simulink model "ZynqBF_2tx_fpga"  (R2018b)
settings: Solver=FixedStepDiscrete  StartTime=0.0  StopTime=10.0  RelTol=1e-3
undefined symbols (not defined in the file or in its folder): gs1_i, gs1_q, gs2_i, gs2_q
libraries: hdlsllib x22, simulink x20, dsphdlfiltering x4
settings Model: DataTypeOverride=Off  Creator=jason  LastModifiedBy=jason
settings DataIOCC: SaveOutput=off  SaveTime=off
settings OptimizationCC: BlockReduction=off  ConditionallyExecuteInputs=off  DefaultParameterBehavior=Inlined
settings DebuggingCC: AlgebraicLoopMsg=error  SingleTaskRateTransMsg=error  ParameterPrecisionLossMsg=none  StrictBusMsg=ErrorOnBusTreatedAsVector
settings HardwareCC: ProdBitPerPointer=32  ProdBitPerSizeT=32  ProdBitPerPtrDiffT=32  ProdLargestAtomicFloat=None  ProdIntDivRoundTo=Undefined  ProdEndianess=Unspecified  ProdWordSize=32  ProdHWDeviceType=ASIC/FPGA->ASIC/FPGA  ProdEqTarget=off
settings SFSimCC: SimUseLocalCustomCode=off
settings RTWCC: RTWUseLocalCustomCode=off
settings CodeAppCC: StateflowObjectComments=on
settings GRTTargetCC: TargetLangStandard=C89/C90 (ANSI)

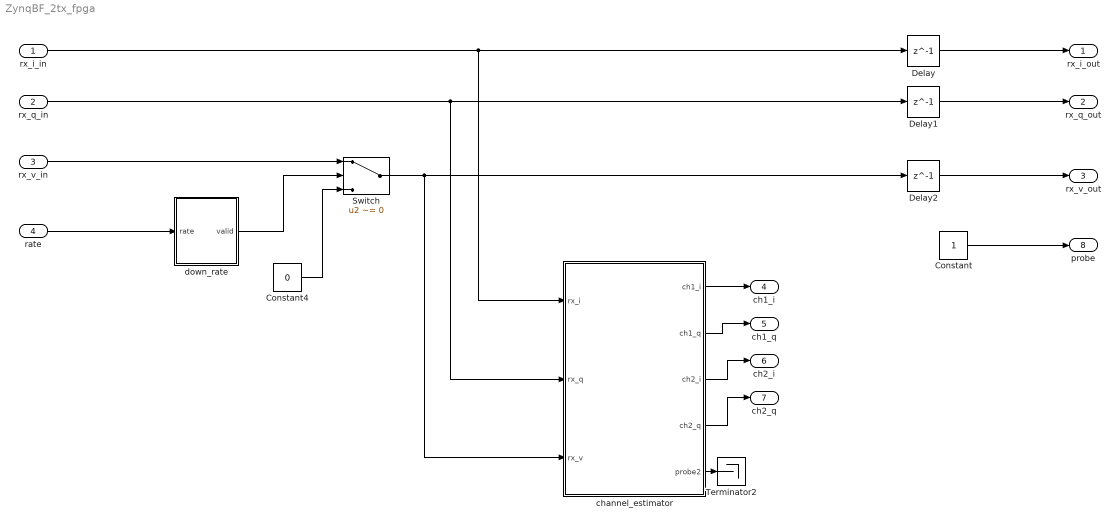
== system ZynqBF_2tx_fpga ==
  rx_i_in : Inport  OutDataTypeStr=fixdt(1,16,15)  SampleTime=1
  rx_q_in : Inport  Port=2  OutDataTypeStr=fixdt(1,16,15)  SampleTime=1
  rx_v_in : Inport  Port=3  OutDataTypeStr=boolean  SampleTime=1
  rate : Inport  Port=4  OutDataTypeStr=uint16  SampleTime=1
  Constant : Constant  OutDataTypeStr=uint16  SampleTime=-1
  Constant4 : Constant  Value=0  OutDataTypeStr=boolean  SampleTime=-1
  Delay : Delay  DelayLength=1
  Delay1 : Delay  DelayLength=1
  Delay2 : Delay  DelayLength=1
  Switch : Switch  Criteria=u2 ~= 0
  Terminator2 : Terminator
  channel_estimator : Subsystem  TreatAsAtomicUnit=on
  down_rate : Subsystem  TreatAsAtomicUnit=on
  rx_i_out : Outport  OutDataTypeStr=fixdt(1,16,15)
  rx_q_out : Outport  Port=2  OutDataTypeStr=fixdt(1,16,15)
  rx_v_out : Outport  Port=3  OutDataTypeStr=boolean  LockScale=on
  ch1_i : Outport  Port=4  OutDataTypeStr=fixdt(1,16,15)
  ch1_q : Outport  Port=5  OutDataTypeStr=fixdt(1,16,15)
  ch2_i : Outport  Port=6  OutDataTypeStr=fixdt(1,16,15)
  ch2_q : Outport  Port=7  OutDataTypeStr=fixdt(1,16,15)
  probe : Outport  Port=8
  wires:
  rate/1 -> down_rate/1(rate)
  rx_i_in/1 -> channel_estimator/1(rx_i), Delay/1
  rx_q_in/1 -> channel_estimator/2(rx_q), Delay1/1
  down_rate/1(valid) -> Switch/2
  rx_v_in/1 -> Switch/1
  Switch/1 -> channel_estimator/3(rx_v), Delay2/1
  Constant4/1 -> Switch/3
  Delay/1 -> rx_i_out/1
  Delay1/1 -> rx_q_out/1
  Delay2/1 -> rx_v_out/1
  channel_estimator/1(ch1_i) -> ch1_i/1
  channel_estimator/2(ch1_q) -> ch1_q/1
  channel_estimator/3(ch2_i) -> ch2_i/1
  channel_estimator/4(ch2_q) -> ch2_q/1
  channel_estimator/5(probe2) -> Terminator2/1
  Constant/1 -> probe/1

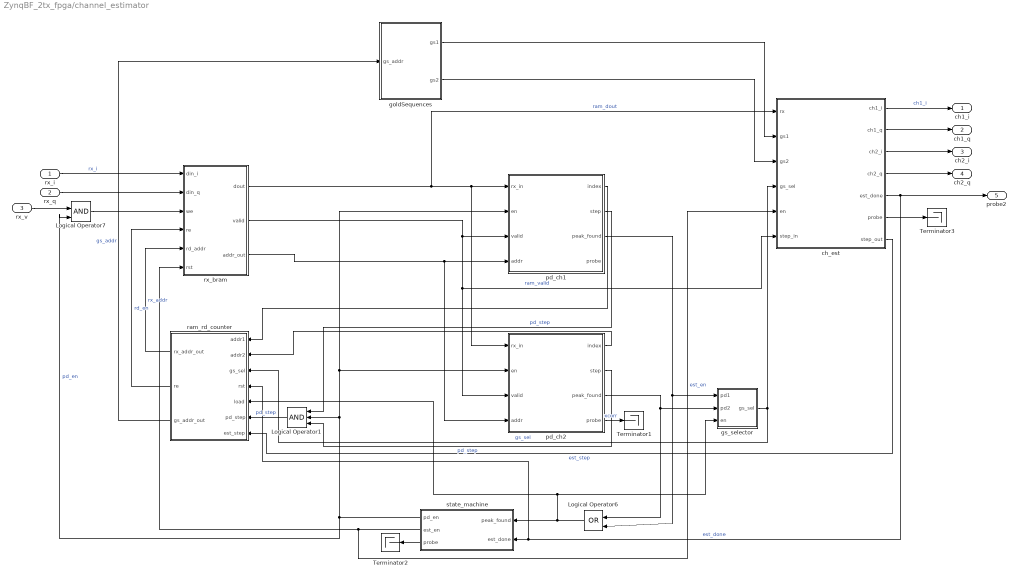
== system ZynqBF_2tx_fpga/channel_estimator ==
  rx_i : Inport
  rx_q : Inport  Port=2
  rx_v : Inport  Port=3
  Logical Operator1 : Logic  Inputs=3  IconShape=distinctive  AllPortsSameDT=off  OutDataTypeStr=boolean
  Logical Operator6 : Logic  Operator=OR  IconShape=distinctive  AllPortsSameDT=off  OutDataTypeStr=boolean
  Logical Operator7 : Logic  IconShape=distinctive  AllPortsSameDT=off  OutDataTypeStr=boolean
  Terminator1 : Terminator
  Terminator2 : Terminator
  Terminator3 : Terminator
  ch_est : Subsystem
  goldSequences : Subsystem
  gs_selector : Subsystem
  pd_ch1 : Subsystem
  pd_ch2 : Subsystem
  ram_rd_counter : Subsystem
  rx_bram : Subsystem
  state_machine : Subsystem
  ch1_i : Outport
  ch1_q : Outport  Port=2
  ch2_i : Outport  Port=3
  ch2_q : Outport  Port=4
  probe2 : Outport  Port=5
  wires:
  rx_q/1 -> rx_bram/2(din_q)
  rx_i/1 -> rx_bram/1(din_i)  "rx_i"
  Logical Operator7/1 -> rx_bram/3(we)
  pd_ch1/2(step) -> Logical Operator1/1  "pd_step"
  rx_bram/1(dout) -> ch_est/1(rx), pd_ch1/1(rx_in), pd_ch2/1(rx_in)  "ram_dout"
  goldSequences/1(gs1) -> ch_est/2(gs1)
  state_machine/1(pd_en) -> pd_ch1/2(en), pd_ch2/2(en), Logical Operator1/2, Logical Operator7/2  "pd_en"
  Logical Operator6/1 -> ram_rd_counter/5(load), gs_selector/3(en), state_machine/1(peak_found)
  ch_est/5(est_done) -> ram_rd_counter/4(rst), state_machine/2(est_done), probe2/1  "est_done"
  rx_v/1 -> Logical Operator7/1
  goldSequences/2(gs2) -> ch_est/3(gs2)
  pd_ch2/3(peak_found) -> Logical Operator6/1, gs_selector/2(pd2)
  pd_ch1/3(peak_found) -> Logical Operator6/2, gs_selector/1(pd1)
  gs_selector/1(gs_sel) -> ch_est/4(gs_sel), ram_rd_counter/3(gs_sel)  "gs_sel"
  ch_est/1(ch1_i) -> ch1_i/1  "ch1_i"
  ch_est/2(ch1_q) -> ch1_q/1
  ch_est/3(ch2_i) -> ch2_i/1
  ch_est/4(ch2_q) -> ch2_q/1
  rx_bram/2(valid) -> pd_ch1/3(valid), pd_ch2/3(valid), ch_est/6(step_in)  "ram_valid"
  Logical Operator1/1 -> ram_rd_counter/6(pd_step)  "pd_step"
  ram_rd_counter/1(rx_addr_out) -> rx_bram/5(rd_addr)  "rx_addr"
  ram_rd_counter/2(re) -> rx_bram/4(re)  "rd_en"
  state_machine/2(est_en) -> rx_bram/6(rst), ch_est/5(en)  "est_en"
  rx_bram/3(addr_out) -> pd_ch1/4(addr), pd_ch2/4(addr)
  ram_rd_counter/3(gs_addr_out) -> goldSequences/1(gs_addr)  "gs_addr"
  ch_est/7(step_out) -> ram_rd_counter/7(est_step)  "est_step"
  pd_ch2/2(step) -> Logical Operator1/3  "pd_step"
  pd_ch1/1(index) -> ram_rd_counter/1(addr1)
  pd_ch2/1(index) -> ram_rd_counter/2(addr2)
  pd_ch2/4(probe) -> Terminator1/1  "xcorr"
  state_machine/3(probe) -> Terminator2/1
  ch_est/6(probe) -> Terminator3/1

== system ZynqBF_2tx_fpga/down_rate ==
  rate : Inport
  HDL Counter : hdlsllib/Sources/HDL Counter  CountType=Free running  CountInit=0  CountStep=1  CountMax=25  CountFromType=Initial value  CountFrom=0  CountResetPort=on  CountLoadPort=off  CountEnbPort=off  CountDirPort=off  CountDataType=Unsigned  CountWordLen=8  CountFracLen=0  CountSampTime=1
      settings: SourceProductBaseCode=HD
  Relational Operator : RelationalOperator  OutDataTypeStr=boolean  RndMeth=Nearest
  valid : Outport
  wires:
  HDL Counter/1 -> Relational Operator/1
  Relational Operator/1 -> valid/1, HDL Counter/1
  rate/1 -> Relational Operator/2

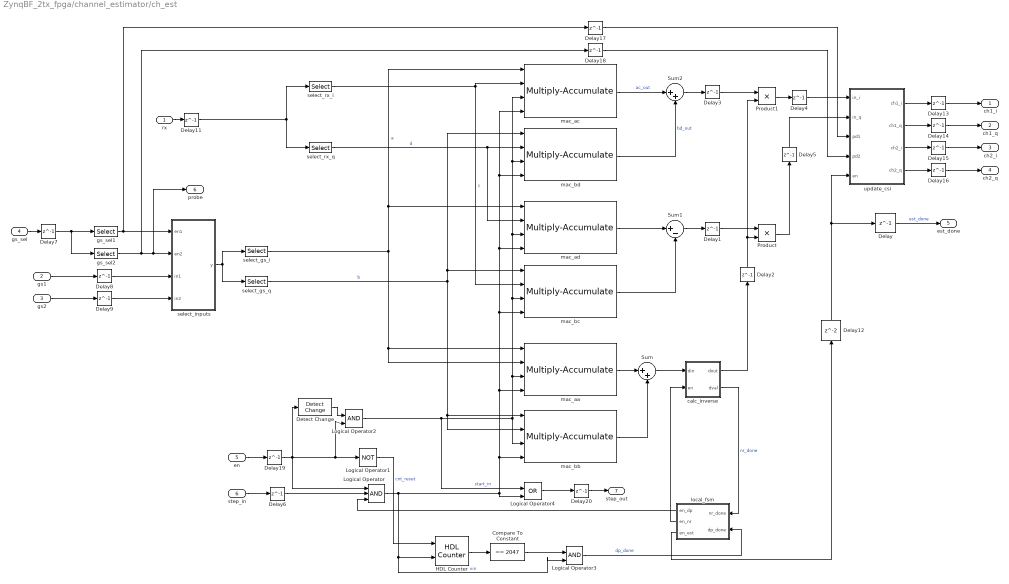
== system ZynqBF_2tx_fpga/channel_estimator/ch_est ==
  rx : Inport
  gs1 : Inport  Port=2
  gs2 : Inport  Port=3
  gs_sel : Inport  Port=4
  en : Inport  Port=5
  step_in : Inport  Port=6
  Compare To Constant : simulink/Logic and Bit Operations/Compare To Constant  relop===  const=2047  OutDataTypeStr=boolean
  Delay{,1..9,11,13..20} (19 alike) : Delay  DelayLength=1
  Delay12 : Delay
  Detect Change : simulink/Logic and Bit Operations/Detect Change  vinit=0  OutDataTypeStr=boolean
  HDL Counter : hdlsllib/Sources/HDL Counter  CountType=Count limited  CountInit=0  CountStep=1  CountMax=2047  CountFromType=Initial value  CountFrom=0  CountResetPort=on  CountLoadPort=off  CountEnbPort=on  CountDirPort=off  CountDataType=Unsigned  CountWordLen=16  CountFracLen=0  CountSampTime=-1
      settings: SourceProductBaseCode=HD
  Logical Operator : Logic  Inputs=3  IconShape=distinctive  AllPortsSameDT=off  OutDataTypeStr=boolean
  Logical Operator1 : Logic  Operator=NOT  IconShape=distinctive  AllPortsSameDT=off  OutDataTypeStr=boolean
  Logical Operator2 : Logic  IconShape=distinctive  AllPortsSameDT=off  OutDataTypeStr=boolean
  Logical Operator3 : Logic  IconShape=distinctive  AllPortsSameDT=off  OutDataTypeStr=boolean
  Logical Operator4 : Logic  Operator=OR  IconShape=distinctive  AllPortsSameDT=off  OutDataTypeStr=boolean
  Product : Product  OutDataTypeStr=fixdt(1,16,15)
  Product1 : Product  OutDataTypeStr=fixdt(1,16,15)
  Sum : Sum  Inputs=|++  OutDataTypeStr=fixdt(1,32,16)
  Sum1 : Sum  Inputs=|+-  OutDataTypeStr=fixdt(1,32,16)
  Sum2 : Sum  Inputs=|++  OutDataTypeStr=fixdt(1,32,16)
  calc_inverse : Subsystem
  gs_sel1 : Selector  IndexMode=Zero-based  InputPortWidth=2  IndexOptions=Index vector (dialog)  Indices=[0]  OutputSizes=1
  gs_sel2 : Selector  IndexMode=Zero-based  InputPortWidth=2  IndexOptions=Index vector (dialog)  Indices=[1]  OutputSizes=1
  local_fsm : Subsystem
  mac_aa : hdlsllib/HDL Operations/Multiply-Accumulate  opMode=Streaming - using Start and End ports  initValueSetting=Dialog  initValue=0  initValueSetting2=Dialog  initValue2=0  initValueSetting3=Dialog  initValue3=0  num_samples=2048  RndMeth2=Floor  RndMeth3=Floor  datatype2=fixdt(1,32,16)  datatype3=Inherit: Inherit via back propagation  validOut=off  endInandOut=off  startOut=off  countOut=off  dim=-1  DoSatur=off  parallel=off
      settings: SourceProductName=HDL Coder  SourceProductBaseCode=HD
  mac_ac : hdlsllib/HDL Operations/Multiply-Accumulate  opMode=Streaming - using Start and End ports  initValueSetting=Dialog  initValue=0  initValueSetting2=Dialog  initValue2=0  initValueSetting3=Dialog  initValue3=0  num_samples=2048  RndMeth2=Floor  RndMeth3=Floor  datatype2=fixdt(1,32,16)  datatype3=Inherit: Inherit via back propagation  validOut=off  endInandOut=off  startOut=off  countOut=off  dim=-1  DoSatur=off  parallel=off
      settings: SourceProductName=HDL Coder  SourceProductBaseCode=HD
  mac_ad : hdlsllib/HDL Operations/Multiply-Accumulate  opMode=Streaming - using Start and End ports  initValueSetting=Dialog  initValue=0  initValueSetting2=Dialog  initValue2=0  initValueSetting3=Dialog  initValue3=0  num_samples=2048  RndMeth2=Floor  RndMeth3=Floor  datatype2=fixdt(1,32,16)  datatype3=Inherit: Inherit via back propagation  validOut=off  endInandOut=off  startOut=off  countOut=off  dim=-1  DoSatur=off  parallel=off
      settings: SourceProductName=HDL Coder  SourceProductBaseCode=HD
  mac_bb : hdlsllib/HDL Operations/Multiply-Accumulate  opMode=Streaming - using Start and End ports  initValueSetting=Dialog  initValue=0  initValueSetting2=Dialog  initValue2=0  initValueSetting3=Dialog  initValue3=0  num_samples=2048  RndMeth2=Floor  RndMeth3=Floor  datatype2=fixdt(1,32,16)  datatype3=Inherit: Inherit via back propagation  validOut=off  endInandOut=off  startOut=off  countOut=off  dim=-1  DoSatur=off  parallel=off
      settings: SourceProductName=HDL Coder  SourceProductBaseCode=HD
  mac_bc : hdlsllib/HDL Operations/Multiply-Accumulate  opMode=Streaming - using Start and End ports  initValueSetting=Dialog  initValue=0  initValueSetting2=Dialog  initValue2=0  initValueSetting3=Dialog  initValue3=0  num_samples=2048  RndMeth2=Floor  RndMeth3=Floor  datatype2=fixdt(1,32,16)  datatype3=Inherit: Inherit via back propagation  validOut=off  endInandOut=off  startOut=off  countOut=off  dim=-1  DoSatur=off  parallel=off
      settings: SourceProductName=HDL Coder  SourceProductBaseCode=HD
  mac_bd : hdlsllib/HDL Operations/Multiply-Accumulate  opMode=Streaming - using Start and End ports  initValueSetting=Dialog  initValue=0  initValueSetting2=Dialog  initValue2=0  initValueSetting3=Dialog  initValue3=0  num_samples=2048  RndMeth2=Floor  RndMeth3=Floor  datatype2=fixdt(1,32,16)  datatype3=Inherit: Inherit via back propagation  validOut=off  endInandOut=off  startOut=off  countOut=off  dim=-1  DoSatur=off  parallel=off
      settings: SourceProductName=HDL Coder  SourceProductBaseCode=HD
  select_gs_i : Selector  IndexMode=Zero-based  InputPortWidth=2  IndexOptions=Index vector (dialog)  Indices=[0]  OutputSizes=1
  select_gs_q : Selector  IndexMode=Zero-based  InputPortWidth=2  IndexOptions=Index vector (dialog)  Indices=[1]  OutputSizes=1
  select_inputs : MATLAB Function  TreatAsAtomicUnit=on
  select_rx_i : Selector  IndexMode=Zero-based  InputPortWidth=2  IndexOptions=Index vector (dialog)  Indices=[0]  OutputSizes=1
  select_rx_q : Selector  IndexMode=Zero-based  InputPortWidth=2  IndexOptions=Index vector (dialog)  Indices=[1]  OutputSizes=1
  update_csi : Subsystem
  ch1_i : Outport
  ch1_q : Outport  Port=2
  ch2_i : Outport  Port=3
  ch2_q : Outport  Port=4
  est_done : Outport  Port=5
  probe : Outport  Port=6
  step_out : Outport  Port=7
  wires:
  gs_sel/1 -> Delay7/1
  select_rx_i/1 -> mac_bc/2, mac_ac/2  "c"
  select_rx_q/1 -> mac_ad/2, mac_bd/2  "d"
  Logical Operator/1 -> Logical Operator4/2, mac_ac/4, mac_bd/4, mac_ad/4, mac_bc/4, mac_aa/4, mac_bb/4, Logical Operator3/2, HDL Counter/2  "vin"
  gs1/1 -> Delay8/1
  gs2/1 -> Delay9/1
  select_inputs/1(y) -> select_gs_q/1, select_gs_i/1
  mac_ad/1 -> Sum1/1
  mac_bc/1 -> Sum1/2
  mac_ac/1 -> Sum2/1  "ac_out"
  mac_bd/1 -> Sum2/2  "bd_out"
  step_in/1 -> Delay6/1
  local_fsm/1(en_dp) -> Logical Operator/3
  Sum/1 -> calc_inverse/1(din)
  calc_inverse/2(dval) -> local_fsm/1(nr_done)  "nr_done"
  local_fsm/2(en_nr) -> calc_inverse/2(en)
  calc_inverse/1(dout) -> Delay2/1
  Sum1/1 -> Delay1/1
  Sum2/1 -> Delay3/1
  local_fsm/3(en_est) -> Delay12/1
  Product1/1 -> Delay4/1
  Product/1 -> Delay5/1
  update_csi/1(ch1_i) -> Delay13/1
  update_csi/2(ch1_q) -> Delay14/1
  update_csi/3(ch2_i) -> Delay15/1
  update_csi/4(ch2_q) -> Delay16/1
  Delay/1 -> est_done/1  "est_done"
  rx/1 -> Delay11/1
  Delay11/1 -> select_rx_i/1, select_rx_q/1
  Delay2/1 -> Product1/2, Product/2
  Delay1/1 -> Product/1
  Delay3/1 -> Product1/1
  Delay4/1 -> update_csi/1(in_i)
  Delay5/1 -> update_csi/2(in_q)
  Delay6/1 -> Logical Operator/2
  Delay8/1 -> select_inputs/3(in1)
  Delay9/1 -> select_inputs/4(in2)
  Delay12/1 -> Delay/1, update_csi/5(en)
  Delay13/1 -> ch1_i/1
  Delay14/1 -> ch1_q/1
  Delay15/1 -> ch2_i/1
  Delay16/1 -> ch2_q/1
  Delay7/1 -> gs_sel2/1, gs_sel1/1
  gs_sel2/1 -> Delay18/1, probe/1, select_inputs/2(en2)
  gs_sel1/1 -> Delay17/1, select_inputs/1(en1)
  Delay17/1 -> update_csi/3(pd1)
  Delay18/1 -> update_csi/4(pd2)
  select_gs_i/1 -> mac_aa/1, mac_aa/2, mac_ac/1, mac_ad/1  "a"
  select_gs_q/1 -> mac_bb/2, mac_bb/1, mac_bd/1, mac_bc/1  "b"
  en/1 -> Delay19/1
  Logical Operator1/1 -> HDL Counter/1  "cnt_reset"
  Delay19/1 -> Logical Operator/1, Detect Change/1, Logical Operator2/2, Logical Operator1/1
  Detect Change/1 -> Logical Operator2/1
  Logical Operator2/1 -> Logical Operator4/1, mac_bb/3, mac_aa/3, mac_bc/3, mac_ad/3, mac_bd/3, mac_ac/3  "start_in"
  HDL Counter/1 -> Compare To Constant/1
  mac_aa/1 -> Sum/1
  mac_bb/1 -> Sum/2
  Delay20/1 -> step_out/1
  Compare To Constant/1 -> Logical Operator3/1
  Logical Operator3/1 -> local_fsm/2(dp_done)  "dp_done"
  Logical Operator4/1 -> Delay20/1

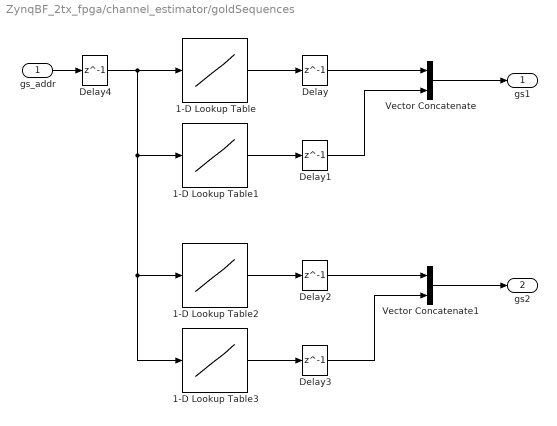
== system ZynqBF_2tx_fpga/channel_estimator/goldSequences ==
  gs_addr : Inport
  1-D Lookup Table : Lookup_n-D  NumberOfTableDimensions=1  LookupTableObject=''  BreakpointsForDimension1=[0:2047]  BreakpointsForDimension1FirstPoint=10  BreakpointsForDimension2FirstPoint=10  BreakpointsForDimension1Spacing=12  BreakpointsForDimension2Spacing=12  IndexSearchMethod=Evenly spaced points  Table=gs1_i  InterpMethod=Flat  DiagnosticForOutOfRangeInput=Error  InternalRulePriority=Speed  OutDataTypeStr=fixdt(1,16,15)  RndMeth=Simplest  InputSameDT=on
  1-D Lookup Table1 : Lookup_n-D  NumberOfTableDimensions=1  LookupTableObject=''  BreakpointsForDimension1=[0:2047]  BreakpointsForDimension1FirstPoint=10  BreakpointsForDimension2FirstPoint=10  BreakpointsForDimension1Spacing=12  BreakpointsForDimension2Spacing=12  IndexSearchMethod=Evenly spaced points  Table=gs1_q  InterpMethod=Flat  DiagnosticForOutOfRangeInput=Error  InternalRulePriority=Speed  OutDataTypeStr=fixdt(1,16,15)  RndMeth=Simplest  InputSameDT=on
  1-D Lookup Table2 : Lookup_n-D  NumberOfTableDimensions=1  LookupTableObject=''  BreakpointsForDimension1=[0:2047]  BreakpointsForDimension1FirstPoint=10  BreakpointsForDimension2FirstPoint=10  BreakpointsForDimension1Spacing=12  BreakpointsForDimension2Spacing=12  IndexSearchMethod=Evenly spaced points  Table=gs2_i  InterpMethod=Flat  DiagnosticForOutOfRangeInput=Error  InternalRulePriority=Speed  OutDataTypeStr=fixdt(1,16,15)  RndMeth=Simplest  InputSameDT=on
  1-D Lookup Table3 : Lookup_n-D  NumberOfTableDimensions=1  LookupTableObject=''  BreakpointsForDimension1=[0:2047]  BreakpointsForDimension1FirstPoint=10  BreakpointsForDimension2FirstPoint=10  BreakpointsForDimension1Spacing=12  BreakpointsForDimension2Spacing=12  IndexSearchMethod=Evenly spaced points  Table=gs2_q  InterpMethod=Flat  DiagnosticForOutOfRangeInput=Error  InternalRulePriority=Speed  OutDataTypeStr=fixdt(1,16,15)  RndMeth=Simplest  InputSameDT=on
  Delay{,1..4} (5 alike) : Delay  DelayLength=1
  Vector Concatenate : Concatenate
  Vector Concatenate1 : Concatenate
  gs1 : Outport
  gs2 : Outport  Port=2
  wires:
  1-D Lookup Table/1 -> Delay/1
  1-D Lookup Table1/1 -> Delay1/1
  1-D Lookup Table3/1 -> Delay3/1
  1-D Lookup Table2/1 -> Delay2/1
  Vector Concatenate/1 -> gs1/1
  Vector Concatenate1/1 -> gs2/1
  Delay/1 -> Vector Concatenate/1
  Delay1/1 -> Vector Concatenate/2
  Delay2/1 -> Vector Concatenate1/1
  Delay3/1 -> Vector Concatenate1/2
  gs_addr/1 -> Delay4/1
  Delay4/1 -> 1-D Lookup Table3/1, 1-D Lookup Table2/1, 1-D Lookup Table1/1, 1-D Lookup Table/1

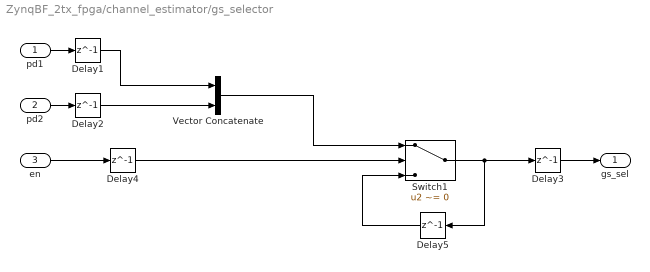
== system ZynqBF_2tx_fpga/channel_estimator/gs_selector ==
  pd1 : Inport
  pd2 : Inport  Port=2
  en : Inport  Port=3
  Delay{1..5} (5 alike) : Delay  DelayLength=1
  Switch1 : Switch  Criteria=u2 ~= 0
  Vector Concatenate : Concatenate
  gs_sel : Outport
  wires:
  pd2/1 -> Delay2/1
  en/1 -> Delay4/1
  pd1/1 -> Delay1/1
  Delay2/1 -> Vector Concatenate/2
  Delay1/1 -> Vector Concatenate/1
  Delay3/1 -> gs_sel/1
  Switch1/1 -> Delay3/1, Delay5/1
  Delay4/1 -> Switch1/2
  Vector Concatenate/1 -> Switch1/1
  Delay5/1 -> Switch1/3

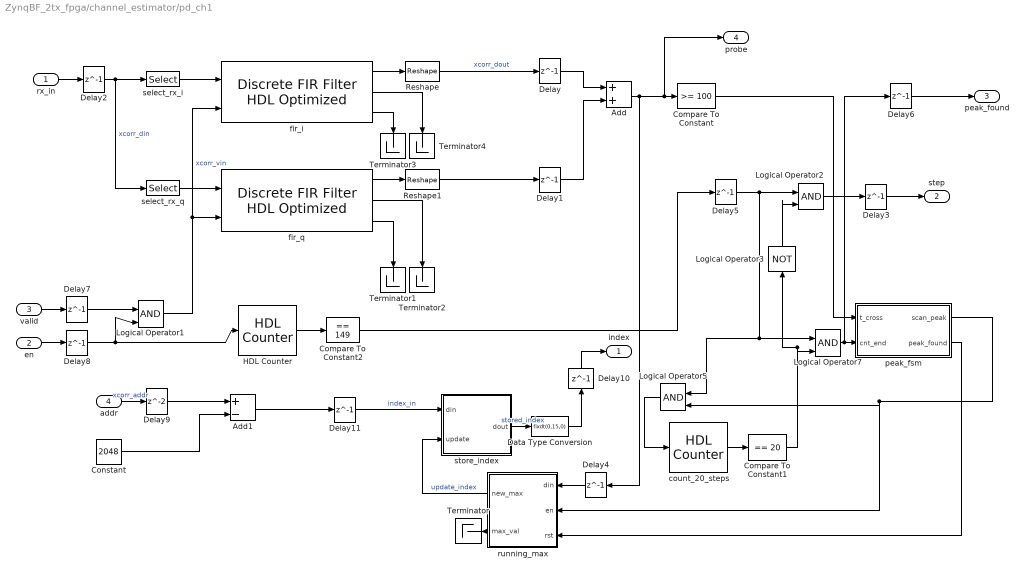
== system ZynqBF_2tx_fpga/channel_estimator/pd_ch1 ==
  rx_in : Inport
  en : Inport  Port=2
  valid : Inport  Port=3
  addr : Inport  Port=4
  Add : Sum  OutDataTypeStr=fixdt(1,32,16)
  Add1 : Sum  Inputs=+-  OutDataTypeStr=int16
  Compare To Constant : simulink/Logic and Bit Operations/Compare To Constant  relop=>=  const=100  OutDataTypeStr=boolean
  Compare To Constant1 : simulink/Logic and Bit Operations/Compare To Constant  relop===  const=20  OutDataTypeStr=boolean
  Compare To Constant2 : simulink/Logic and Bit Operations/Compare To Constant  relop===  const=149  OutDataTypeStr=boolean
  Constant : Constant  Value=2048  OutDataTypeStr=uint16  SampleTime=-1
  Data Type Conversion : DataTypeConversion  OutDataTypeStr=fixdt(0,15,0)
  Delay{,1..8,10..11} (11 alike) : Delay  DelayLength=1
  Delay9 : Delay
  HDL Counter : hdlsllib/Sources/HDL Counter  CountType=Count limited  CountInit=0  CountStep=1  CountMax=149  CountFromType=Initial value  CountFrom=0  CountResetPort=off  CountLoadPort=off  CountEnbPort=on  CountDirPort=off  CountDataType=Unsigned  CountWordLen=8  CountFracLen=0  CountSampTime=1
      settings: SourceProductBaseCode=HD
  Logical Operator{1..2,5,7} (4 alike) : Logic  IconShape=distinctive  AllPortsSameDT=off  OutDataTypeStr=boolean
  Logical Operator3 : Logic  Operator=NOT  IconShape=distinctive  AllPortsSameDT=off  OutDataTypeStr=boolean
  Reshape : Reshape
  Reshape1 : Reshape
  Terminator{,1..4} (5 alike) : Terminator
  count_20_steps : hdlsllib/Sources/HDL Counter  CountType=Count limited  CountInit=0  CountStep=1  CountMax=20  CountFromType=Initial value  CountFrom=0  CountResetPort=off  CountLoadPort=off  CountEnbPort=on  CountDirPort=off  CountDataType=Unsigned  CountWordLen=8  CountFracLen=0  CountSampTime=1
      settings: SourceProductBaseCode=HD
  fir_i : dsphdlfiltering/Discrete FIR Filter HDL Optimized  Numerator=fliplr(gs1_i')  FilterStructure=Direct form systolic  Sharing=on  SharingFactor=128  SimulateUsing=Code generation  roundingMode=Floor  overflowMode=off  CoefficientsDataTypeStr=Inherit: Same word length as input  CoefficientsMin=[]  CoefficientsMax=[]  OutputMin=[]  OutputMax=[]  ResetInputPort=off  HDLGlobalReset=off
      settings: SourceProductName=DSP System Toolbox  SourceProductBaseCode=DS
  fir_q : dsphdlfiltering/Discrete FIR Filter HDL Optimized  Numerator=fliplr(gs1_q')  FilterStructure=Direct form systolic  Sharing=on  SharingFactor=128  SimulateUsing=Code generation  roundingMode=Floor  overflowMode=off  CoefficientsDataTypeStr=Inherit: Same word length as input  CoefficientsMin=[]  CoefficientsMax=[]  OutputMin=[]  OutputMax=[]  ResetInputPort=off  HDLGlobalReset=off
      settings: SourceProductName=DSP System Toolbox  SourceProductBaseCode=DS
  peak_fsm : Subsystem
  running_max : Subsystem
  select_rx_i : Selector  IndexMode=Zero-based  InputPortWidth=2  IndexOptions=Index vector (dialog)  Indices=[0]  OutputSizes=1
  select_rx_q : Selector  IndexMode=Zero-based  InputPortWidth=2  IndexOptions=Index vector (dialog)  Indices=[1]  OutputSizes=1
  store_index : Subsystem
  index : Outport
  step : Outport  Port=2
  peak_found : Outport  Port=3
  probe : Outport  Port=4
  wires:
  Data Type Conversion/1 -> Delay10/1
  rx_in/1 -> Delay2/1
  fir_i/1 -> Reshape/1
  Reshape1/1 -> Delay1/1
  Delay1/1 -> Add/2
  Delay/1 -> Add/1
  Add/1 -> probe/1, Compare To Constant/1, Delay4/1
  Compare To Constant/1 -> peak_fsm/1(t_cross)
  Compare To Constant2/1 -> Delay5/1
  peak_fsm/1(scan_peak) -> running_max/2(en), Logical Operator5/2
  Logical Operator5/1 -> count_20_steps/1
  count_20_steps/1 -> Compare To Constant1/1
  Compare To Constant1/1 -> Logical Operator3/1, Logical Operator7/2
  Logical Operator7/1 -> Delay6/1, peak_fsm/2(cnt_end)
  peak_fsm/2(peak_found) -> running_max/3(rst)
  Delay4/1 -> running_max/1(din)
  running_max/2(max_val) -> Terminator/1
  en/1 -> Delay8/1
  Delay5/1 -> Logical Operator2/1, Logical Operator5/1, Logical Operator7/1
  Delay6/1 -> peak_found/1
  Reshape/1 -> Delay/1  "xcorr_dout"
  HDL Counter/1 -> Compare To Constant2/1
  fir_q/1 -> Reshape1/1
  valid/1 -> Delay7/1
  Logical Operator1/1 -> fir_i/2, fir_q/2  "xcorr_vin"
  Delay7/1 -> Logical Operator1/1
  Delay8/1 -> Logical Operator1/2, HDL Counter/1
  addr/1 -> Delay9/1  "xcorr_addr"
  Constant/1 -> Add1/2
  Delay9/1 -> Add1/1
  Add1/1 -> Delay11/1
  running_max/1(new_max) -> store_index/2(update)  "update_index"
  Delay11/1 -> store_index/1(din)  "index_in"
  store_index/1(dout) -> Data Type Conversion/1  "stored_index"
  Delay10/1 -> index/1
  Delay2/1 -> select_rx_q/1, select_rx_i/1  "xcorr_din"
  select_rx_i/1 -> fir_i/1
  select_rx_q/1 -> fir_q/1
  Logical Operator2/1 -> Delay3/1
  Logical Operator3/1 -> Logical Operator2/2
  Delay3/1 -> step/1
  fir_q/3 -> Terminator1/1
  fir_q/2 -> Terminator2/1
  fir_i/3 -> Terminator3/1
  fir_i/2 -> Terminator4/1

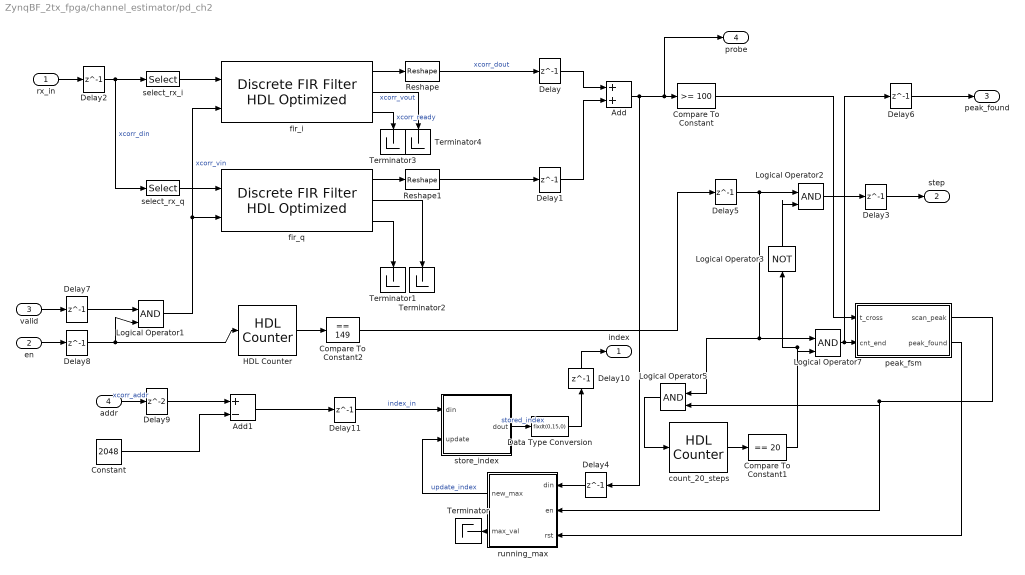
== system ZynqBF_2tx_fpga/channel_estimator/pd_ch2 ==
  rx_in : Inport
  en : Inport  Port=2
  valid : Inport  Port=3
  addr : Inport  Port=4
  Add : Sum  OutDataTypeStr=fixdt(1,32,16)
  Add1 : Sum  Inputs=+-  OutDataTypeStr=int16
  Compare To Constant : simulink/Logic and Bit Operations/Compare To Constant  relop=>=  const=100  OutDataTypeStr=boolean
  Compare To Constant1 : simulink/Logic and Bit Operations/Compare To Constant  relop===  const=20  OutDataTypeStr=boolean
  Compare To Constant2 : simulink/Logic and Bit Operations/Compare To Constant  relop===  const=149  OutDataTypeStr=boolean
  Constant : Constant  Value=2048  OutDataTypeStr=uint16  SampleTime=-1
  Data Type Conversion : DataTypeConversion  OutDataTypeStr=fixdt(0,15,0)
  Delay{,1..8,10..11} (11 alike) : Delay  DelayLength=1
  Delay9 : Delay
  HDL Counter : hdlsllib/Sources/HDL Counter  CountType=Count limited  CountInit=0  CountStep=1  CountMax=149  CountFromType=Initial value  CountFrom=0  CountResetPort=off  CountLoadPort=off  CountEnbPort=on  CountDirPort=off  CountDataType=Unsigned  CountWordLen=8  CountFracLen=0  CountSampTime=1
      settings: SourceProductBaseCode=HD
  Logical Operator{1..2,5,7} (4 alike) : Logic  IconShape=distinctive  AllPortsSameDT=off  OutDataTypeStr=boolean
  Logical Operator3 : Logic  Operator=NOT  IconShape=distinctive  AllPortsSameDT=off  OutDataTypeStr=boolean
  Reshape : Reshape
  Reshape1 : Reshape
  Terminator{,1..4} (5 alike) : Terminator
  count_20_steps : hdlsllib/Sources/HDL Counter  CountType=Count limited  CountInit=0  CountStep=1  CountMax=20  CountFromType=Initial value  CountFrom=0  CountResetPort=off  CountLoadPort=off  CountEnbPort=on  CountDirPort=off  CountDataType=Unsigned  CountWordLen=8  CountFracLen=0  CountSampTime=1
      settings: SourceProductBaseCode=HD
  fir_i : dsphdlfiltering/Discrete FIR Filter HDL Optimized  Numerator=fliplr(gs2_i')  FilterStructure=Direct form systolic  Sharing=on  SharingFactor=128  SimulateUsing=Code generation  roundingMode=Floor  overflowMode=off  CoefficientsDataTypeStr=Inherit: Same word length as input  CoefficientsMin=[]  CoefficientsMax=[]  OutputMin=[]  OutputMax=[]  ResetInputPort=off  HDLGlobalReset=off
      settings: SourceProductName=DSP System Toolbox  SourceProductBaseCode=DS
  fir_q : dsphdlfiltering/Discrete FIR Filter HDL Optimized  Numerator=fliplr(gs2_q')  FilterStructure=Direct form systolic  Sharing=on  SharingFactor=128  SimulateUsing=Code generation  roundingMode=Floor  overflowMode=off  CoefficientsDataTypeStr=Inherit: Same word length as input  CoefficientsMin=[]  CoefficientsMax=[]  OutputMin=[]  OutputMax=[]  ResetInputPort=off  HDLGlobalReset=off
      settings: SourceProductName=DSP System Toolbox  SourceProductBaseCode=DS
  peak_fsm : Subsystem
  running_max : Subsystem
  select_rx_i : Selector  IndexMode=Zero-based  InputPortWidth=2  IndexOptions=Index vector (dialog)  Indices=[0]  OutputSizes=1
  select_rx_q : Selector  IndexMode=Zero-based  InputPortWidth=2  IndexOptions=Index vector (dialog)  Indices=[1]  OutputSizes=1
  store_index : Subsystem
  index : Outport
  step : Outport  Port=2
  peak_found : Outport  Port=3
  probe : Outport  Port=4
  wires:
  Delay3/1 -> step/1
  Logical Operator3/1 -> Logical Operator2/2
  Logical Operator2/1 -> Delay3/1
  select_rx_q/1 -> fir_q/1
  select_rx_i/1 -> fir_i/1
  Delay2/1 -> select_rx_i/1, select_rx_q/1  "xcorr_din"
  Delay10/1 -> index/1
  store_index/1(dout) -> Data Type Conversion/1  "stored_index"
  Delay11/1 -> store_index/1(din)  "index_in"
  running_max/1(new_max) -> store_index/2(update)  "update_index"
  Add1/1 -> Delay11/1
  Delay9/1 -> Add1/1
  Constant/1 -> Add1/2
  addr/1 -> Delay9/1  "xcorr_addr"
  Delay8/1 -> HDL Counter/1, Logical Operator1/2
  Delay7/1 -> Logical Operator1/1
  Logical Operator1/1 -> fir_q/2, fir_i/2  "xcorr_vin"
  valid/1 -> Delay7/1
  fir_q/1 -> Reshape1/1
  HDL Counter/1 -> Compare To Constant2/1
  Reshape/1 -> Delay/1  "xcorr_dout"
  Delay6/1 -> peak_found/1
  Delay5/1 -> Logical Operator7/1, Logical Operator5/1, Logical Operator2/1
  en/1 -> Delay8/1
  running_max/2(max_val) -> Terminator/1
  Delay4/1 -> running_max/1(din)
  peak_fsm/2(peak_found) -> running_max/3(rst)
  Logical Operator7/1 -> peak_fsm/2(cnt_end), Delay6/1
  Compare To Constant1/1 -> Logical Operator7/2, Logical Operator3/1
  count_20_steps/1 -> Compare To Constant1/1
  Logical Operator5/1 -> count_20_steps/1
  peak_fsm/1(scan_peak) -> Logical Operator5/2, running_max/2(en)
  Compare To Constant2/1 -> Delay5/1
  Compare To Constant/1 -> peak_fsm/1(t_cross)
  Add/1 -> Delay4/1, Compare To Constant/1, probe/1
  Delay/1 -> Add/1
  Delay1/1 -> Add/2
  Reshape1/1 -> Delay1/1
  fir_i/1 -> Reshape/1
  rx_in/1 -> Delay2/1
  Data Type Conversion/1 -> Delay10/1
  fir_q/3 -> Terminator1/1
  fir_q/2 -> Terminator2/1
  fir_i/3 -> Terminator3/1  "xcorr_ready"
  fir_i/2 -> Terminator4/1  "xcorr_vout"

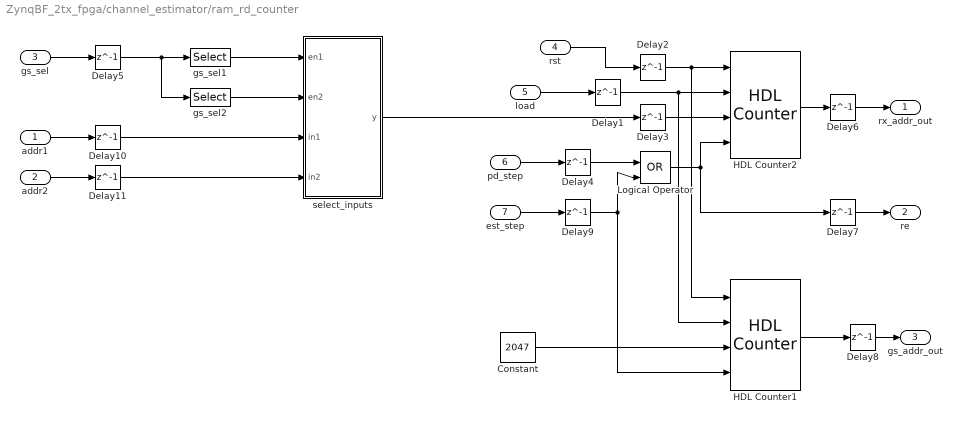
== system ZynqBF_2tx_fpga/channel_estimator/ram_rd_counter ==
  addr1 : Inport
  addr2 : Inport  Port=2
  gs_sel : Inport  Port=3
  rst : Inport  Port=4
  load : Inport  Port=5
  pd_step : Inport  Port=6
  est_step : Inport  Port=7
  Constant : Constant  Value=2047  OutDataTypeStr=Inherit: Inherit via back propagation  SampleTime=-1
  Delay{1..5,7,9..11} (9 alike) : Delay  DelayLength=1
  Delay6 : Delay  DelayLength=1  InitialCondition=0
  Delay8 : Delay  DelayLength=1  InitialCondition=0
  HDL Counter1 : hdlsllib/Sources/HDL Counter  CountType=Count limited  CountInit=0  CountStep=1  CountMax=2047  CountFromType=Initial value  CountFrom=0  CountResetPort=on  CountLoadPort=on  CountEnbPort=on  CountDirPort=off  CountDataType=Unsigned  CountWordLen=11  CountFracLen=0  CountSampTime=1
      settings: SourceProductBaseCode=HD
  HDL Counter2 : hdlsllib/Sources/HDL Counter  CountType=Count limited  CountInit=0  CountStep=1  CountMax=32767  CountFromType=Initial value  CountFrom=0  CountResetPort=on  CountLoadPort=on  CountEnbPort=on  CountDirPort=off  CountDataType=Unsigned  CountWordLen=15  CountFracLen=0  CountSampTime=1
      settings: SourceProductBaseCode=HD
  Logical Operator : Logic  Operator=OR  IconShape=distinctive  AllPortsSameDT=off  OutDataTypeStr=boolean
  gs_sel1 : Selector  IndexMode=Zero-based  InputPortWidth=2  IndexOptions=Index vector (dialog)  Indices=[0]  OutputSizes=1
  gs_sel2 : Selector  IndexMode=Zero-based  InputPortWidth=2  IndexOptions=Index vector (dialog)  Indices=[1]  OutputSizes=1
  select_inputs : MATLAB Function  TreatAsAtomicUnit=on
  rx_addr_out : Outport
  re : Outport  Port=2
  gs_addr_out : Outport  Port=3
  wires:
  rst/1 -> Delay2/1
  load/1 -> Delay1/1
  Logical Operator/1 -> HDL Counter2/4, Delay7/1
  select_inputs/1(y) -> Delay3/1
  HDL Counter2/1 -> Delay6/1
  pd_step/1 -> Delay4/1
  Delay2/1 -> HDL Counter1/1, HDL Counter2/1
  Delay1/1 -> HDL Counter1/2, HDL Counter2/2
  Delay3/1 -> HDL Counter2/3
  Delay4/1 -> Logical Operator/1
  Delay9/1 -> HDL Counter1/4, Logical Operator/2
  Delay6/1 -> rx_addr_out/1
  Delay7/1 -> re/1
  HDL Counter1/1 -> Delay8/1
  Delay8/1 -> gs_addr_out/1
  est_step/1 -> Delay9/1
  Constant/1 -> HDL Counter1/3
  gs_sel/1 -> Delay5/1
  Delay5/1 -> gs_sel2/1, gs_sel1/1
  gs_sel1/1 -> select_inputs/1(en1)
  gs_sel2/1 -> select_inputs/2(en2)
  addr1/1 -> Delay10/1
  addr2/1 -> Delay11/1
  Delay10/1 -> select_inputs/3(in1)
  Delay11/1 -> select_inputs/4(in2)

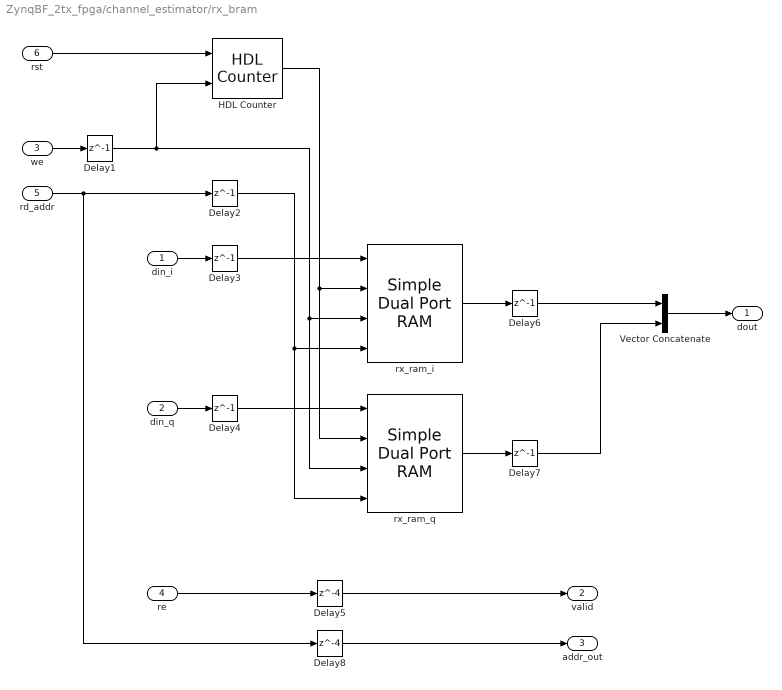
== system ZynqBF_2tx_fpga/channel_estimator/rx_bram ==
  din_i : Inport  OutDataTypeStr=fixdt(1,16,15)
  din_q : Inport  Port=2  OutDataTypeStr=fixdt(1,16,15)
  we : Inport  Port=3  OutDataTypeStr=boolean
  re : Inport  Port=4  OutDataTypeStr=boolean
  rd_addr : Inport  Port=5
  rst : Inport  Port=6  OutDataTypeStr=boolean
  Delay{1..4,6..7} (6 alike) : Delay  DelayLength=1
  Delay5 : Delay  DelayLength=4
  Delay8 : Delay  DelayLength=4
  HDL Counter : hdlsllib/Sources/HDL Counter  CountType=Count limited  CountInit=1  CountStep=1  CountMax=32767  CountFromType=Initial value  CountFrom=1  CountResetPort=on  CountLoadPort=off  CountEnbPort=on  CountDirPort=off  CountDataType=Unsigned  CountWordLen=15  CountFracLen=0  CountSampTime=1
      settings: SourceProductBaseCode=HD
  Vector Concatenate : Concatenate
  rx_ram_i : hdlsllib/HDL RAMs/Simple Dual Port RAM  ram_size=15
      settings: SourceProductName=HDL Coder  SourceProductBaseCode=HD
  rx_ram_q : hdlsllib/HDL RAMs/Simple Dual Port RAM  ram_size=15
      settings: SourceProductName=HDL Coder  SourceProductBaseCode=HD
  dout : Outport
  valid : Outport  Port=2
  addr_out : Outport  Port=3
  wires:
  we/1 -> Delay1/1
  din_q/1 -> Delay4/1
  rx_ram_q/1 -> Delay7/1
  din_i/1 -> Delay3/1
  rd_addr/1 -> Delay8/1, Delay2/1
  rx_ram_i/1 -> Delay6/1
  HDL Counter/1 -> rx_ram_q/2, rx_ram_i/2
  Delay1/1 -> HDL Counter/2, rx_ram_q/3, rx_ram_i/3
  Delay2/1 -> rx_ram_q/4, rx_ram_i/4
  Delay3/1 -> rx_ram_i/1
  Delay4/1 -> rx_ram_q/1
  re/1 -> Delay5/1
  Delay5/1 -> valid/1
  rst/1 -> HDL Counter/1
  Delay7/1 -> Vector Concatenate/2
  Delay8/1 -> addr_out/1
  Vector Concatenate/1 -> dout/1
  Delay6/1 -> Vector Concatenate/1

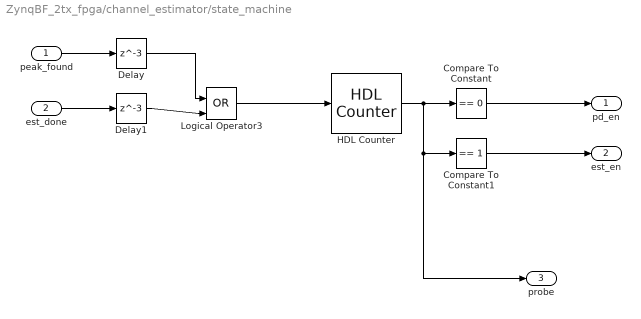
== system ZynqBF_2tx_fpga/channel_estimator/state_machine ==
  peak_found : Inport
  est_done : Inport  Port=2
  Compare To Constant : simulink/Logic and Bit Operations/Compare To Constant  relop===  const=0  OutDataTypeStr=boolean
  Compare To Constant1 : simulink/Logic and Bit Operations/Compare To Constant  relop===  const=1  OutDataTypeStr=boolean
  Delay : Delay  DelayLength=3
  Delay1 : Delay  DelayLength=3
  HDL Counter : hdlsllib/Sources/HDL Counter  CountType=Count limited  CountInit=0  CountStep=1  CountMax=1  CountFromType=Initial value  CountFrom=0  CountResetPort=off  CountLoadPort=off  CountEnbPort=on  CountDirPort=off  CountDataType=Unsigned  CountWordLen=8  CountFracLen=0  CountSampTime=1
      settings: SourceProductBaseCode=HD
  Logical Operator3 : Logic  Operator=OR  IconShape=distinctive  AllPortsSameDT=off  OutDataTypeStr=boolean
  pd_en : Outport
  est_en : Outport  Port=2
  probe : Outport  Port=3
  wires:
  est_done/1 -> Delay1/1
  HDL Counter/1 -> probe/1, Compare To Constant1/1, Compare To Constant/1
  peak_found/1 -> Delay/1
  Logical Operator3/1 -> HDL Counter/1
  Delay/1 -> Logical Operator3/1
  Delay1/1 -> Logical Operator3/2
  Compare To Constant/1 -> pd_en/1
  Compare To Constant1/1 -> est_en/1

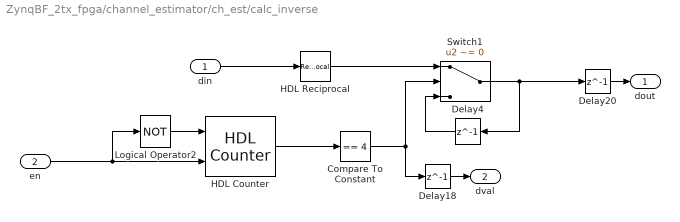
== system ZynqBF_2tx_fpga/channel_estimator/ch_est/calc_inverse ==
  din : Inport
  en : Inport  Port=2
  Compare To Constant : simulink/Logic and Bit Operations/Compare To Constant  relop===  const=4  OutDataTypeStr=boolean
  Delay18 : Delay  DelayLength=1
  Delay20 : Delay  DelayLength=1
  Delay4 : Delay  DelayLength=1
  HDL Counter : hdlsllib/Sources/HDL Counter  CountType=Count limited  CountInit=0  CountStep=1  CountMax=9  CountFromType=Initial value  CountFrom=0  CountResetPort=on  CountLoadPort=off  CountEnbPort=on  CountDirPort=off  CountDataType=Unsigned  CountWordLen=8  CountFracLen=0  CountSampTime=1
      settings: SourceProductBaseCode=HD
  HDL Reciprocal : Reciprocal  NumberOfIterations=5
  Logical Operator2 : Logic  Operator=NOT  IconShape=distinctive  AllPortsSameDT=off  OutDataTypeStr=boolean
  Switch1 : Switch  Criteria=u2 ~= 0
  dout : Outport
  dval : Outport  Port=2
  wires:
  Logical Operator2/1 -> HDL Counter/1
  Compare To Constant/1 -> Switch1/2, Delay18/1
  HDL Reciprocal/1 -> Switch1/1
  en/1 -> Logical Operator2/1, HDL Counter/2
  HDL Counter/1 -> Compare To Constant/1
  Delay18/1 -> dval/1
  Delay20/1 -> dout/1
  din/1 -> HDL Reciprocal/1
  Switch1/1 -> Delay20/1, Delay4/1
  Delay4/1 -> Switch1/3

== system ZynqBF_2tx_fpga/channel_estimator/ch_est/local_fsm ==
  nr_done : Inport
  dp_done : Inport  Port=2
  Compare To Constant : simulink/Logic and Bit Operations/Compare To Constant  relop===  const=0  OutDataTypeStr=boolean
  Compare To Constant1 : simulink/Logic and Bit Operations/Compare To Constant  relop===  const=1  OutDataTypeStr=boolean
  Compare To Constant2 : simulink/Logic and Bit Operations/Compare To Constant  relop===  const=2  OutDataTypeStr=boolean
  HDL Counter : hdlsllib/Sources/HDL Counter  CountType=Count limited  CountInit=0  CountStep=1  CountMax=2  CountFromType=Initial value  CountFrom=0  CountResetPort=off  CountLoadPort=off  CountEnbPort=on  CountDirPort=off  CountDataType=Unsigned  CountWordLen=8  CountFracLen=0  CountSampTime=1
      settings: SourceProductBaseCode=HD
  Logical Operator : Logic  Operator=OR  Inputs=3  IconShape=distinctive  AllPortsSameDT=off  OutDataTypeStr=boolean
  en_dp : Outport
  en_nr : Outport  Port=2
  en_est : Outport  Port=3
  wires:
  Logical Operator/1 -> HDL Counter/1
  dp_done/1 -> Logical Operator/1
  nr_done/1 -> Logical Operator/2
  HDL Counter/1 -> Compare To Constant/1, Compare To Constant2/1, Compare To Constant1/1
  Compare To Constant/1 -> en_dp/1
  Compare To Constant1/1 -> en_nr/1
  Compare To Constant2/1 -> Logical Operator/3, en_est/1

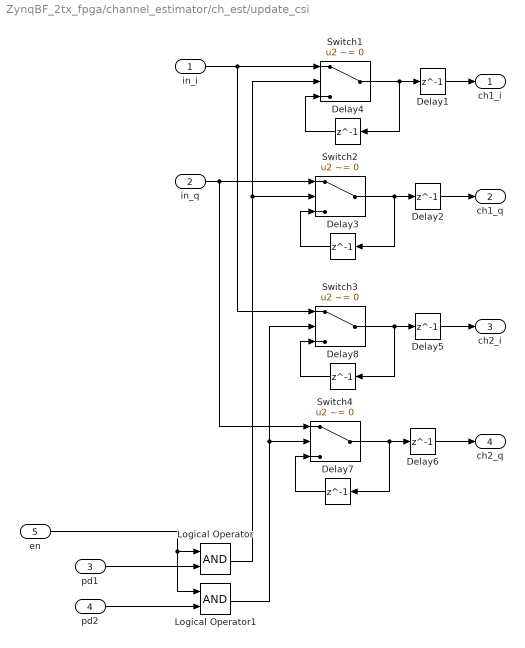
== system ZynqBF_2tx_fpga/channel_estimator/ch_est/update_csi ==
  in_i : Inport
  in_q : Inport  Port=2
  pd1 : Inport  Port=3
  pd2 : Inport  Port=4
  en : Inport  Port=5
  Delay{1..8} (8 alike) : Delay  DelayLength=1
  Logical Operator : Logic  AllPortsSameDT=off  OutDataTypeStr=boolean
  Logical Operator1 : Logic  AllPortsSameDT=off  OutDataTypeStr=boolean
  Switch{1..4} (4 alike) : Switch  Criteria=u2 ~= 0
  ch1_i : Outport
  ch1_q : Outport  Port=2
  ch2_i : Outport  Port=3
  ch2_q : Outport  Port=4
  wires:
  pd1/1 -> Logical Operator/2
  en/1 -> Logical Operator1/1, Logical Operator/1
  Logical Operator/1 -> Switch1/2, Switch2/2
  pd2/1 -> Logical Operator1/2
  Switch1/1 -> Delay1/1, Delay4/1
  Delay4/1 -> Switch1/3
  Delay1/1 -> ch1_i/1
  Delay2/1 -> ch1_q/1
  Switch2/1 -> Delay2/1, Delay3/1
  Delay3/1 -> Switch2/3
  Switch3/1 -> Delay5/1, Delay8/1
  in_i/1 -> Switch3/1, Switch1/1
  in_q/1 -> Switch4/1, Switch2/1
  Delay7/1 -> Switch4/3
  Delay8/1 -> Switch3/3
  Delay5/1 -> ch2_i/1
  Switch4/1 -> Delay6/1, Delay7/1
  Delay6/1 -> ch2_q/1
  Logical Operator1/1 -> Switch3/2, Switch4/2

== system ZynqBF_2tx_fpga/channel_estimator/pd_ch1/peak_fsm ==
  t_cross : Inport
  cnt_end : Inport  Port=2
  Compare To Constant : simulink/Logic and Bit Operations/Compare To Constant  relop===  const=1  OutDataTypeStr=boolean
  Compare To Constant1 : simulink/Logic and Bit Operations/Compare To Constant  relop===  const=0  OutDataTypeStr=boolean
  Compare To Constant2 : simulink/Logic and Bit Operations/Compare To Constant  relop===  const=2  OutDataTypeStr=boolean
  HDL Counter : hdlsllib/Sources/HDL Counter  CountType=Count limited  CountInit=0  CountStep=1  CountMax=3  CountFromType=Initial value  CountFrom=0  CountResetPort=off  CountLoadPort=off  CountEnbPort=on  CountDirPort=off  CountDataType=Unsigned  CountWordLen=8  CountFracLen=0  CountSampTime=1
      settings: SourceProductBaseCode=HD
  Logical Operator : Logic  IconShape=distinctive  AllPortsSameDT=off  OutDataTypeStr=boolean
  Logical Operator1 : Logic  Operator=OR  Inputs=3  IconShape=distinctive  AllPortsSameDT=off  OutDataTypeStr=boolean
  scan_peak : Outport
  peak_found : Outport  Port=2
  wires:
  HDL Counter/1 -> Compare To Constant2/1, Compare To Constant/1, Compare To Constant1/1
  Compare To Constant1/1 -> Logical Operator/2
  t_cross/1 -> Logical Operator/1
  Compare To Constant/1 -> scan_peak/1
  Logical Operator1/1 -> HDL Counter/1
  Logical Operator/1 -> Logical Operator1/3
  cnt_end/1 -> Logical Operator1/2
  Compare To Constant2/1 -> Logical Operator1/1, peak_found/1

== system ZynqBF_2tx_fpga/channel_estimator/pd_ch1/running_max ==
  din : Inport
  en : Inport  Port=2
  rst : Inport  Port=3
  Constant : Constant  Value=0  OutDataTypeStr=fixdt(1,32,16)  SampleTime=-1
  Delay4 : Delay  DelayLength=1
  Relational Operator : RelationalOperator  Operator=>  OutDataTypeStr=boolean  RndMeth=Nearest
  reset_max : Switch  Criteria=u2 ~= 0
  store_max : Switch  Criteria=u2 ~= 0
  update_max : Logic  IconShape=distinctive  AllPortsSameDT=off  OutDataTypeStr=boolean
  new_max : Outport
  max_val : Outport  Port=2
  wires:
  reset_max/1 -> Delay4/1
  Constant/1 -> reset_max/1
  Relational Operator/1 -> update_max/2
  store_max/1 -> reset_max/3
  Delay4/1 -> store_max/3, max_val/1, Relational Operator/2
  en/1 -> update_max/1
  din/1 -> store_max/1, Relational Operator/1
  rst/1 -> reset_max/2
  update_max/1 -> new_max/1, store_max/2  "update_max_p"

== system ZynqBF_2tx_fpga/channel_estimator/pd_ch1/store_index ==
  din : Inport
  update : Inport  Port=2
  Delay{1..2,4..5} (4 alike) : Delay  DelayLength=1
  Switch : Switch  Criteria=u2 ~= 0
  dout : Outport
  wires:
  Delay5/1 -> Switch/3
  update/1 -> Delay1/1
  din/1 -> Delay2/1
  Switch/1 -> Delay4/1, Delay5/1
  Delay2/1 -> Switch/1
  Delay1/1 -> Switch/2
  Delay4/1 -> dout/1

== system ZynqBF_2tx_fpga/channel_estimator/pd_ch2/peak_fsm ==
  t_cross : Inport
  cnt_end : Inport  Port=2
  Compare To Constant : simulink/Logic and Bit Operations/Compare To Constant  relop===  const=1  OutDataTypeStr=boolean
  Compare To Constant1 : simulink/Logic and Bit Operations/Compare To Constant  relop===  const=0  OutDataTypeStr=boolean
  Compare To Constant2 : simulink/Logic and Bit Operations/Compare To Constant  relop===  const=2  OutDataTypeStr=boolean
  HDL Counter : hdlsllib/Sources/HDL Counter  CountType=Count limited  CountInit=0  CountStep=1  CountMax=3  CountFromType=Initial value  CountFrom=0  CountResetPort=off  CountLoadPort=off  CountEnbPort=on  CountDirPort=off  CountDataType=Unsigned  CountWordLen=8  CountFracLen=0  CountSampTime=1
      settings: SourceProductBaseCode=HD
  Logical Operator : Logic  IconShape=distinctive  AllPortsSameDT=off  OutDataTypeStr=boolean
  Logical Operator1 : Logic  Operator=OR  Inputs=3  IconShape=distinctive  AllPortsSameDT=off  OutDataTypeStr=boolean
  scan_peak : Outport
  peak_found : Outport  Port=2
  wires:
  Compare To Constant2/1 -> peak_found/1, Logical Operator1/1
  cnt_end/1 -> Logical Operator1/2
  Logical Operator/1 -> Logical Operator1/3
  Logical Operator1/1 -> HDL Counter/1
  Compare To Constant/1 -> scan_peak/1
  t_cross/1 -> Logical Operator/1
  Compare To Constant1/1 -> Logical Operator/2
  HDL Counter/1 -> Compare To Constant1/1, Compare To Constant/1, Compare To Constant2/1

== system ZynqBF_2tx_fpga/channel_estimator/pd_ch2/running_max ==
  din : Inport
  en : Inport  Port=2
  rst : Inport  Port=3
  Constant : Constant  Value=0  OutDataTypeStr=fixdt(1,32,16)  SampleTime=-1
  Delay4 : Delay  DelayLength=1
  Relational Operator : RelationalOperator  Operator=>  OutDataTypeStr=boolean  RndMeth=Nearest
  reset_max : Switch  Criteria=u2 ~= 0
  store_max : Switch  Criteria=u2 ~= 0
  update_max : Logic  IconShape=distinctive  AllPortsSameDT=off  OutDataTypeStr=boolean
  new_max : Outport
  max_val : Outport  Port=2
  wires:
  update_max/1 -> store_max/2, new_max/1  "update_max_p"
  rst/1 -> reset_max/2
  din/1 -> Relational Operator/1, store_max/1
  en/1 -> update_max/1
  Delay4/1 -> Relational Operator/2, max_val/1, store_max/3
  store_max/1 -> reset_max/3
  Relational Operator/1 -> update_max/2
  Constant/1 -> reset_max/1
  reset_max/1 -> Delay4/1

== system ZynqBF_2tx_fpga/channel_estimator/pd_ch2/store_index ==
  din : Inport
  update : Inport  Port=2
  Delay{1..2,4..5} (4 alike) : Delay  DelayLength=1
  Switch : Switch  Criteria=u2 ~= 0
  dout : Outport
  wires:
  Delay4/1 -> dout/1
  Delay1/1 -> Switch/2
  Delay2/1 -> Switch/1
  Switch/1 -> Delay5/1, Delay4/1
  din/1 -> Delay2/1
  update/1 -> Delay1/1
  Delay5/1 -> Switch/3

== matlab function ZynqBF_2tx_fpga/channel_estimator/ram_rd_counter/select_inputs ==
  data: en1 input; y output; en2 input; in1 input; in2 input
function y = fcn(en1, en2, in1, in2)
%#codegen

if (en1 && en2)
    y = zeros(1,1,'like',in1);
elseif (en1)
    y = in1;
elseif (en2)
    y = in2;
else
    y = zeros(1,1,'like',in1);
end

== matlab function ZynqBF_2tx_fpga/channel_estimator/ch_est/select_inputs ==
  data: en1 input; y output; en2 input; in1 input; in2 input
function y = fcn(en1, en2, in1, in2)
%#codegen

if (en1 && en2)
    y = zeros(2,1,'like',in1);
elseif (en1)
    y = in1;
elseif (en2)
    y = in2;
else
    y = zeros(2,1,'like',in1);
end
